simulink model "Second_connected_val"  (R2015b)
settings: Solver=ode14x  StartTime=0.0  StopTime=10.22  FixedStep=0.02  RelTol=1e-3
values from neighbouring files (symbols this model uses):
  c = b1(i)+ D    [backup_connected.m]    (also in connected_La_zero.m = b1(j2) + D; connected_current_speed.m = b2(j2) + D; connected_current_speed_La_zero.m = b2(j2) + D; fmin.m = b + D)
  J = b1(i)+ Jm    [backup_connected.m]    (also in connected_La_zero.m = b2(i)+ Jm; connected_current_speed.m; connected_current_speed_La_zero.m; fmin.m = a + Jm)
  Ke = 7.06*10^-2    (= 0.0706)    [Project3_matlab.m]    (also in backup_connected.m; connected_La_zero.m; connected_current_speed.m; connected_current_speed_La_zero.m)
  Kt = 7.06*10^-2    (= 0.0706)    [Project3_matlab.m]    (also in backup_connected.m; connected_La_zero.m; connected_current_speed.m; connected_current_speed_La_zero.m)
  La = 0.87*10^-3    (= 0.00087)    [Project3_matlab.m]    (also in backup_connected.m; connected_La_zero.m = 0; connected_current_speed.m; connected_current_speed_La_zero.m = 0)
  Ra = 0.59    [Project3_matlab.m]    (also in backup_connected.m; connected_La_zero.m; connected_current_speed.m; connected_current_speed_La_zero.m)
settings Model: Creator=guilh_000  LastModifiedBy=guilh_000

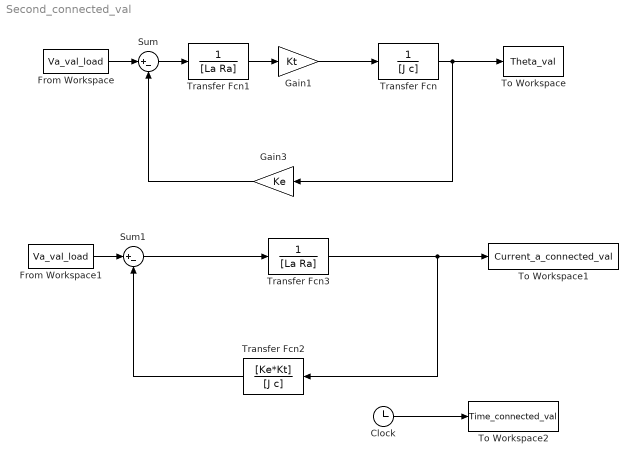
== system Second_connected_val ==
  Clock : Clock
  From Workspace : FromWorkspace  VariableName=Va_val_load  SampleTime=0
  From Workspace1 : FromWorkspace  VariableName=Va_val_load  SampleTime=0
  Gain1 : Gain  Gain=Kt
  Gain3 : Gain  Gain=Ke
  Sum : Sum  Inputs=|+-
  Sum1 : Sum  Inputs=|+-
  To Workspace : ToWorkspace  VariableName=Theta_val  SampleTime=-1
  To Workspace1 : ToWorkspace  VariableName=Current_a_connected_val  SampleTime=-1
  To Workspace2 : ToWorkspace  VariableName=Time_connected_val  SampleTime=-1
  Transfer Fcn : TransferFcn  Denominator=[J c]
  Transfer Fcn1 : TransferFcn  Denominator=[La Ra]
  Transfer Fcn2 : TransferFcn  Numerator=[Ke*Kt]  Denominator=[J c]
  Transfer Fcn3 : TransferFcn  Denominator=[La Ra]
  wires:
  Sum/1 -> Transfer Fcn1/1
  Transfer Fcn1/1 -> Gain1/1
  Gain1/1 -> Transfer Fcn/1
  Transfer Fcn/1 -> Gain3/1, To Workspace/1
  Gain3/1 -> Sum/2
  From Workspace/1 -> Sum/1
  Sum1/1 -> Transfer Fcn3/1
  Transfer Fcn3/1 -> Transfer Fcn2/1, To Workspace1/1
  Transfer Fcn2/1 -> Sum1/2
  From Workspace1/1 -> Sum1/1
  Clock/1 -> To Workspace2/1
